simulink model "truthtable"  (Simulink 7.6)
settings: Solver=FixedStepDiscrete  StartTime=0.0  StopTime=10.0  FixedStep=1  RelTol=1e-3
settings Model: Creator=ksmyth  LastModifiedBy=c2wt
settings OptimizationCC: InitFltsAndDblsToZero=on
settings DebuggingCC: SaveWithParameterizedLinksMsg=none  StrictBusMsg=Warning
settings SFSimCC: SimParseCustomCode=off
settings GRTTargetCC: TargetFcnLib=ansi_tfl_tmw.mat

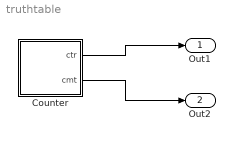
== system truthtable ==
  Counter : Stateflow chart  TreatAsAtomicUnit=on
  Out1 : Outport
  Out2 : Outport  Port=2
  wires:
  Counter/1(ctr) -> Out1/1
  Counter/2(cmt) -> Out2/1

== stateflow chart Counter ==
  state s1
  state y = mod2(x) [function]
    (junction 16) -> (junction 5) [order 2]
    (junction 7) -> (junction 6) : {
        | /* x is odd */
        | y = 0;
        | }
    (junction 16) -> (junction 7) [order 1] : [!aVarTruthTableCondition_1]
    (default) -> (junction 12)
    (junction 12) -> (junction 13) : {
        | /* x is even */
        | aVarTruthTableCondition_1 = (int32(x/2)*2 == x);
        | }
    (junction 13) -> (junction 14) [order 1] : [aVarTruthTableCondition_1]
    (junction 14) -> (junction 15) : {
        | /* 'iseven':x is even */
        | y = 1;
        | }
    (junction 13) -> (junction 16) [order 2]
  (default) -> s1
  (junction 11) -> s1 [order 1] : [ctr < 4] / ctr = ctr+1;
  (junction 11) -> s1 [order 2] : / ctr = -2; cmt = -1;
  s1 -> (junction 8)
  (junction 8) -> (junction 9) : { temp = mod2( ctr ); }
  (junction 9) -> (junction 10) [order 1] : [temp == 1]{cmt = cmt + 1;}
  (junction 9) -> (junction 11) [order 2]
  (junction 10) -> (junction 11)
  data: x function_input int32; y function_output double; aVarTruthTableCondition_1 temporary boolean =0; ctr output double =1; cmt output double; temp local double
  data aVarTruthTableCondition_1 settings: description=x is even
